simulink model "regcontrol_1ph"  (R2018b)
settings: Solver=VariableStepDiscrete  StartTime=0.0  StopTime=20.0  RelTol=1e-3
values from neighbouring files (symbols this model uses):
  BandWidth = Simulink.Parameter    [start.m]
  BaseVoltage = Simulink.Parameter    [start.m]
  CogenEnabled = false    [regcontrol_emulator.m]    (also in start.m = Simulink.Parameter)
  ElementTerminal = 0    [start.m]
  FPTphase = Simulink.Parameter(FPTphases.DEFAULT)    [regcontrol_emulator.m]    (also in start.m = 1)
  InCogenMode = false    [regcontrol_emulator.m]
  InReverseMode = false    [regcontrol_emulator.m]
  IsReversible = Simulink.Parameter    [start.m]
  LDC_Z = Simulink.Parameter    [start.m]
  MaxTap = 1.10    (= 1.1)    [Transformer.m]
  MinTap = 0.90    (= 0.9)    [Transformer.m]
  PTratio = Simulink.Parameter    [start.m]
  R = 0    [start.m]
  RevBand = Simulink.Parameter    [start.m]
  RevVreg = Simulink.Parameter    [start.m]
  TapLimitPerChange = Simulink.Parameter    [start.m]
  UsingRegulatedBus = Simulink.Parameter    [start.m]
  Vlimit = Simulink.Parameter    [start.m]
  Vreg = Simulink.Parameter    [start.m]
  X = 0    [start.m]
undefined symbols (not defined in the file or in its folder): Armed, ControlledTransformerConnection, ControlledTransformerCurrents, ControlledTransformerPowers, ControlledTransformerVoltages, CTRating, DeltaDirection, Handle, IsInverseTime, LastQueue, LookingForward, m, n, NumConductors, NumPhases, PresentTap, RevBackHandle, RevDelay, ReversePending, RevHandle, revLDC_Z, RevPowerThreshold, revR, revX, TapDelay, TapIncrement, TapWinding, TimeDelay, TimeInSec, VTerminal
(part 2 of 2)

== stateflow chart regcontrol_1ph/Queue Handler ==
  settings: enableNonTerminalStates=1
  state Executive [parallel]
    settings: executionOrder=1
    state Asleep
      ex: Status.data = Statuses.READY; % reset status
      INTERNAL_DONE = false;
      EXECUTIVE_DONE = false;
    state DoNearestActions
      state WaitOnPeek
        en: send(QUEUE_PEEK, Internal);
      state WaitOnPop
        en: send(QUEUE_POP, Internal);
      state ErrorNoItems
        en: Status.data = ...
        Statuses.ERROR;
        send(Status);
      (default) -> (junction 302) : % do only those actions with the same delay time as the first action time
          | {q_len_initial = GetQueueSize;
          | PendingActionsCompleted = false; % local for now
          | }
      (junction 302) -> (junction 315) [order 1] : [q_len_initial > 0]
      (junction 302) -> Executive.DoNearestActions.ErrorNoItems [order 2]
      (junction 315) -> WaitOnPeek : {INTERNAL_DONE = false;
          | }
      (junction 301) -> (junction 331) [order 1] : [jj <= q_len_initial]
      (junction 331) -> Executive.DoNearestActions.WaitOnPop : {INTERNAL_DONE = false;}
      WaitOnPeek -> (junction 301) : [INTERNAL_DONE]
          | {ActionTime = Out(QF.Time);
          | jj = 1;}
      Executive.DoNearestActions.WaitOnPop -> (junction 299) : [INTERNAL_DONE]
          | {DoPendingAction.data = ...
          | Out(QF.ActionCode);
          | send(DoPendingAction);}
      (junction 299) -> (junction 301) : {jj = jj + 1;}
      (junction 301) -> (junction 305) [order 2]
      Executive.DoNearestActions.ErrorNoItems -> (junction 300)
      (junction 305) -> (junction 300)
      (junction 300) -> (junction 298) : {EXECUTIVE_DONE = true;}
    state DoAllActions [commented out]
      state WaitOnPop [commented out]
        en: send(QUEUE_POP, Internal);
      state ErrorNoItems [commented out]
        en: Status.data = ...
        Statuses.ERROR;
        send(Status);
      (default) -> (junction 322) [commented out] : {q_len_initial = GetQueueSize;}
      (junction 322) -> (junction 321) [commented out] : [q_len_initial ~= 0]
      (junction 322) -> Executive.DoAllActions.ErrorNoItems [commented out]
      (junction 321) -> (junction 326) [commented out] : {ActionTime = Inf;
          | jj = 1;}
      (junction 326) -> (junction 316) [commented out] : [jj <= q_len_initial]
      (junction 316) -> Executive.DoAllActions.WaitOnPop [commented out] : {INTERNAL_DONE = false;}
      (junction 314) -> (junction 326) [commented out] : {jj = jj + 1;}
      (junction 326) -> (junction 312) [commented out]
      Executive.DoAllActions.WaitOnPop -> (junction 314) [commented out] : [INTERNAL_DONE]
          | %send(DoPendingAction);
      Executive.DoAllActions.ErrorNoItems -> (junction 324) [commented out]
      (junction 312) -> (junction 324) [commented out]
      (junction 324) -> (junction 310) [commented out] : {EXECUTIVE_DONE = true;}
    state Pushing
      en: send(QUEUE_PUSH, Internal);
    state DeletingByHandle
      en: send(QUEUE_DELETE, Internal);
    state Peeking [commented out]
      en: send(QUEUE_PEEK, Internal);
    state Popping [commented out]
      en: send(QUEUE_POP, Internal);
    state ReadyAgain
      Status.data = Statuses.READY;
      send(Status);
    Executive.Asleep -> Executive.DeletingByHandle [order 3] : RegControlAction[RegControlAction.data == ...
        | QueueActions.DELETE]
    Executive.Asleep -> Executive.Peeking [commented out] : QueueAction[QueueAction.data == ...
        | QueueActions.PEEK]
    Executive.Asleep -> Executive.Popping [commented out] : QueueAction[QueueAction.data == ...
        | QueueActions.POP]
    (default) -> Executive.Asleep
    Executive.Asleep -> Executive.Pushing [order 2] : RegControlAction[RegControlAction.data == ...
        | QueueActions.PUSH]
    Executive.Asleep -> DoAllActions [commented out] : QueueAction[QueueAction.data == ...
        | QueueActions.DO_ALL_ACTIONS]
    ReadyAgain -> Executive.Asleep
    Executive.Asleep -> DoNearestActions [order 1] : SolverAction[SolverAction.data == DO_NEAREST_ACTIONS]
    Executive.Pushing -> ReadyAgain : [INTERNAL_DONE]
    Executive.Popping -> ReadyAgain [commented out] : [INTERNAL_DONE]
    Executive.DeletingByHandle -> ReadyAgain : [INTERNAL_DONE]
    Executive.Peeking -> ReadyAgain [commented out] : [INTERNAL_DONE]
    DoAllActions -> ReadyAgain [commented out] : [EXECUTIVE_DONE]
    DoNearestActions -> ReadyAgain : [EXECUTIVE_DONE]
  state Internal [parallel]
    settings: executionOrder=2
    state Asleep
    state DeletingByHandle
      (default) -> (junction 724) : % delete from beginning, t<= ActionTime:
          | {q_len = GetQueueSize;
          | ii = 1;
          | }
      (junction 724) -> (junction 725) [order 1] : [ii <= q_len]
      (junction 725) -> (junction 723)
      (junction 723) -> (junction 726) [order 1] : [GetElemHandle(ii) == uint8(ExternalHandle)]
      (junction 723) -> (junction 722) [order 2]
      (junction 726) -> (junction 710) : {Out = GetElem(ii);
          | ReduceQueue(ii);}
          | % break
      (junction 722) -> (junction 724) : {ii = ii + 1;}
      (junction 724) -> (junction 721) [order 2]
      (junction 710) -> (junction 721)
      (junction 721) -> (junction 706)
      (junction 706) -> (junction 699) [order 1] : [QueueEmpty.data == true]
      (junction 706) -> (junction 709) [order 2]
      (junction 699) -> (junction 704) : {send(QueueEmpty);}
      (junction 704) -> (junction 709)
      (junction 709) -> (junction 700) : {INTERNAL_DONE = true;}
    state Popping
      (default) -> (junction 163) : % delete from beginning, t<= ActionTime:
          | {q_len = GetQueueSize;
          | queue;
          | ii = 1;
          | }
      (junction 163) -> (junction 169) [order 1] : [ii <= q_len]
      (junction 169) -> (junction 157)
      (junction 157) -> (junction 158) [order 1] : [GetElemTime(ii) <= ActionTime]
      (junction 157) -> (junction 164) [order 2]
      (junction 158) -> (junction 159) : {Out = GetElem(ii);
          | ReduceQueue(ii);}
          | % break
      (junction 164) -> (junction 163) : {ii = ii + 1;}
      (junction 163) -> (junction 165) [order 2]
      (junction 159) -> (junction 165)
      (junction 165) -> (junction 640)
      (junction 640) -> (junction 641) [order 1] : [QueueEmpty.data == true]
      (junction 640) -> (junction 642) [order 2]
      (junction 641) -> (junction 643) : {send(QueueEmpty);}
      (junction 643) -> (junction 642)
      (junction 642) -> (junction 644) : {queue;
          | INTERNAL_DONE = true;}
    state Pushing
      (default) -> (junction 136) : % insert into queue right before item of greater or equal execution time
          | {q_cand = In'; % transposition to 1 x 5
          | q_len = GetQueueSize; %size(queue, 3);
          | queue;
          | ii = 1;
          | }
      (junction 136) -> (junction 134) [order 1] : [ii <= q_len]
      (junction 134) -> (junction 145)
      (junction 145) -> (junction 146) [order 1] : [q_cand(1,QF.Time) <= GetElemTime(ii)]
      (junction 145) -> (junction 137) [order 2]
      (junction 146) -> (junction 148) : {ExpandQueue(ii);}
          | % break
      (junction 137) -> (junction 136) : {ii = ii + 1;}
      (junction 136) -> (junction 138) [order 2] : {ExpandQueue(q_len+1);}
      (junction 148) -> (junction 138)
      (junction 138) -> (junction 151) : %{send(DONE_PUSHING, Executive.Pushing);}
          | {queue;
          | INTERNAL_DONE = true;}
    state Peeking
      (default) -> (junction 676) : {q_len = GetQueueSize;
          | }
      (junction 676) -> (junction 677) [order 1] : [q_len >= 1]
      (junction 676) -> (junction 678) [order 2] : {Out = zeros(1,5);}
      (junction 677) -> (junction 679) : {Out = GetElem(1);}
      (junction 679) -> (junction 678)
      (junction 678) -> (junction 689)
      (junction 689) -> (junction 686) [order 1] : [QueueEmpty.data == true]
      (junction 689) -> (junction 687) [order 2]
      (junction 686) -> (junction 684) : {send(QueueEmpty);}
      (junction 684) -> (junction 687)
      (junction 687) -> (junction 685) : {INTERNAL_DONE = true;}
    (default) -> Internal.Asleep
    Internal.Asleep -> Internal.Pushing [order 1] : QUEUE_PUSH
    Internal.Pushing -> Internal.Asleep : [INTERNAL_DONE]
    Internal.Asleep -> Internal.Popping [order 3] : QUEUE_POP
    Internal.Popping -> Internal.Asleep : [INTERNAL_DONE]
    Internal.Asleep -> Internal.Peeking [order 4] : QUEUE_PEEK
    Internal.Peeking -> Internal.Asleep : [INTERNAL_DONE]
    Internal.Asleep -> Internal.DeletingByHandle [order 2] : QUEUE_DELETE
    Internal.DeletingByHandle -> Internal.Asleep : [INTERNAL_DONE]
  state QF % Queue Fields [group]
  state Peeking [parallel] [commented out]
    (default) -> (junction 663) [commented out] : % pop without deletion
        | {q_len = GetQueueSize;
        | ii = 1;
        | }
    (junction 663) -> (junction 666) [commented out] : [ii <= q_len]
    (junction 666) -> (junction 665) [commented out]
    (junction 665) -> (junction 664) [commented out] : [GetElemTime(ii) <= ActionTime]
    (junction 665) -> (junction 662) [commented out]
    (junction 664) -> (junction 659) [commented out] : {Out = GetElem(ii);}
        | % break
    (junction 662) -> (junction 663) [commented out] : {ii = ii + 1;}
    (junction 663) -> (junction 660) [commented out]
    (junction 659) -> (junction 660) [commented out]
    (junction 660) -> (junction 668) [commented out] : {INTERNAL_DONE = true;}
  state qs = GetQueueSize [function]
    (default) -> (junction 649) : {[qs, QueueEmpty.data] = mlGetQueueSize;}
  data: Handle local double =1; Time local double =2; ActionCode local double =5; qs function_output; q_size function_output; qe_data function_output; depth function_input; et function_output; elem function_output; depth function_input; depth function_input; h function_output; depth function_input; depth function_input; RegControlAction input Enum: QueueActions; ExternalHandle input uint8 size=1; SolverAction input Enum: QueueActions; Status output Enum: Statuses; Out output double size=[1 5] =zeros(1,5); queue output double size=[1 5 50]; PendingActionsCompleted local boolean =false; q_cand local double size=[1 5]; In input double size=5; qwriteflag local boolean =false; ii local uint8; jj local uint8; q_len_initial local double; EXECUTIVE_DONE local boolean =false; INTERNAL_DONE local boolean =false;; ActionTime local double; QueueEmpty output boolean =false; PrevQueue input double size=[1 5 50]; DoPendingAction output double =0; q_len output double =0
  events: QUEUE_POP local FUNCTION_CALL_EVENT; QUEUE_PUSH local FUNCTION_CALL_EVENT; QUEUE_PEEK local FUNCTION_CALL_EVENT; QUEUE_DELETE local FUNCTION_CALL_EVENT
  function [q_size, qe_data] = mlGetQueueSize:
    | function [q_size, qe_data] = mlGetQueueSize
    | %     coder.extrinsic('exist');
    | %     eq = zeros(1,1,'double');
    | %     eq = exist('queue');
    | %     if eq == 1 && ~isempty(queue)
    | %         qs = size(queue, 3);
    | %     else % eq ~= 1 || size == 0
    | %         qs = 0;
    | %     end
    |     if ~qwriteflag % can't read intial value of empty queue, so depend on flag
    | %         queue = zeros(1,5);
    | %         if PrevQueue(1,:,1) == zeros(1,5)
    | %             q_size = 0;
    | %             qe_data = true;
    | %         else
    | %             q_size = size(PrevQueue,3);
    | %             queue = PrevQueue;
    | %             qe_data = false;
    | %         end
    |         for qi = 1:size(PrevQueue,3)
    |             if isequal(PrevQueue(1,:,qi), zeros(1,5))
    |                 break;
    |             end
    |         end
    |         q_size = qi - 1; % will be zero for empty queue
    |         if q_size == 0
    |             queue = zeros(1,5);
    |             qe_data = true;
    |         else
    |             queue = PrevQueue(:,:,1:q_size);
    |             qe_data = false;
    |         end
    |         qwriteflag = true;
    |     elseif isequal(queue,zeros(1,5)) % case of empty queue (still 1 element)
    |         q_size = 0;
    |         qe_data = true;
    |         %QueueEmpty.data = true;
    |     else
    |         q_size = size(queue,3);
    |         qe_data = false;
    |         %QueueEmpty.data = false;
    |     end
    | end
  function et = GetElemTime(depth):
    | function et = GetElemTime(depth)
    |     et = zeros(1,1);
    |     if q_len > 0
    |         et = queue(1,QF.Time,ii);
    |     else
    |     end
    | end
  function elem = GetElem(depth):
    | function elem = GetElem(depth)
    |     elem = zeros(1,5);
    |     elem(1,:) = queue(:,:,depth);
    | end
  function h = GetElemHandle(depth):
    | function h = GetElemHandle(depth)
    |     hh = zeros(1,1);
    |     if ~isempty(queue)
    |         hh = queue(1,QF.Handle,ii);        
    |     end
    |     h = cast(hh, 'uint8'); % for comparison with ExternalHandle
    | end
  function ExpandQueue(depth):
    | function ExpandQueue(depth)
    |     rhs = queue(:,:,depth:q_len); % the RHS of the queue
    |     bigger = zeros(1,5,q_len+1);
    |     bigger(:,:,1:(depth-1)) = queue(:,:,1:(depth-1)); % copy LHS
    |     bigger(:,:,depth) = q_cand; % inserting element at end of LHS
    |     %queue(:,:,depth) = q_cand; 
    |     bigger(:,:, (depth+1):(q_len+1)) = rhs; % tack on RHS again
    |     queue = bigger;
    | end
  function ReduceQueue(depth):
    | function ReduceQueue(depth)
    |     rhs = queue(:,:,(depth+1):q_len); % excluding element at depth
    |     smaller = zeros(1,5,q_len-1);
    |     smaller(:,:,1:(depth-1)) = queue(:,:,1:(depth-1)); % lhs, excl. depth
    |     smaller(:,:,depth:(q_len-1)) = rhs; % tack on rhs
    |     if isempty(smaller) || isnan(smaller(1,1,1))
    |         queue = zeros(1,5);
    |     else
    |         queue = smaller;
    |     end
    | end
